simulink library "lib2020a_maxon"  (R2020a)
settings: Solver=VariableStepAuto  StartTime=0.0  StopTime=10.0  RelTol=1e-3
settings Model: Creator=ugurm  LastModifiedBy=Interact Ugur

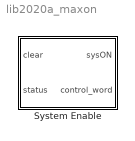
== system lib2020a_maxon ==
  System Enable : Stateflow chart  TreatAsAtomicUnit=on

== stateflow chart lib2020a_maxon/System Enable ==
  settings: sampleTime=0.001
  note: Maxon Motor Driver Device Control
      | v0.5.1
      |
      | Ugur Mengilli
      |
      | Tested on MAXPOS and EPOS4.
  state Device
    entry:   sysON = 0;
    state SwitchOnDisabled
      en: control_word = 6;
    state Fault
      state ClearError
        state SetBit8Low
          en: control_word = 0;
        state ClearFault
          en: control_word = 128;
        SetBit8Low -> ClearFault
      state Wait4ClearSignal
      (default) -> Wait4ClearSignal
    state Ready2SwitchOn
      en: control_word = 15;
    state LimitExceeded
      en: control_word = 0;
    state OperationEnabled
      en: sysON = 1;
      ex: sysON = 0;
    state Init
    Device -> (junction 154) : [hasChanged(clear)]
    Fault -> SwitchOnDisabled : [all(status == 64)]
    SwitchOnDisabled -> Ready2SwitchOn : [all(status == 33)]
    (junction 85) -> Fault [order 1] : [any(status == 8)]
    (junction 72) -> SwitchOnDisabled [order 1] : [all(status == 64)]
    (junction 85) -> (junction 72) [order 2]
    (junction 72) -> Ready2SwitchOn [order 2] : [all(status == 33)]
    LimitExceeded -> (junction 85) : after(1, sec)
    Init -> (junction 85)
    Ready2SwitchOn -> LimitExceeded [order 2] : [any(status == 0)]
    Ready2SwitchOn -> OperationEnabled [order 1] : [all(status == 55)]
    (junction 129) -> LimitExceeded [order 1] : [any(status == 0)]
    (junction 129) -> Init [order 2]
    OperationEnabled -> (junction 129) : [any(status ~= 55)]
    (default) -> Init
    (junction 154) -> SetBit8Low
  data: sysON output double size=1; clear input double size=1; status input double; control_word output uint16 size=1
